simulink model "model"  (R2022a)
settings: Solver=VariableStepAuto  StartTime=0.0  StopTime=0.12  MaxStep=0.0001  RelTol=1e-3
values from neighbouring files (symbols this model uses):
  betta = Mp/wnom    (= 0.600343053173)    [config.m]
  J = J1+J2    (= 0.01)    [config.m]
  Kp = T1/(2*Tmu*Kpr*Kw)    [config.m]
  Kpr = 10    [config.m]
  Kw = u_zad/wnom    (= 0.0857632933105)    [config.m]
  Mc = 0    [config.m]    (also in tasks.m = Mc2)
  T1 = 1/T12(2)    [config.m]
  T2 = 1/T12(1)    [config.m]
  Te = 3.3/1000    (= 0.0033)    [config.m]
  Ti = T1    [config.m]
  Tm = J/betta    (= 0.0166571428571)    [config.m]
  Tmu = Tpr + T2    [config.m]
  Tpr = 0.5/1000    (= 0.0005)    [config.m]
  w_zad = wnom    (= 116.6)    [config.m]    (also in tasks.m = 0)
settings Model: Creator=Vvlad  LastModifiedBy=Vvlad

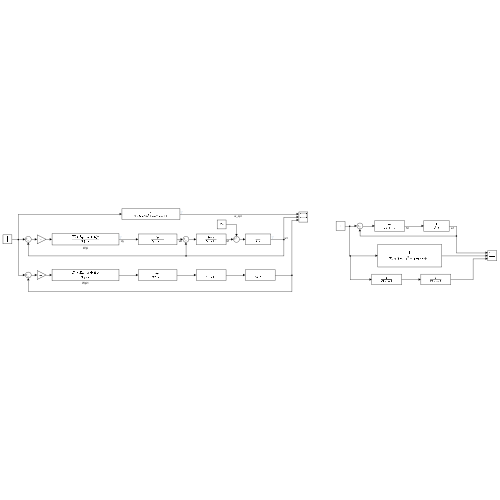
[thumbnail: Simulink's stored preview of the top-level diagram]
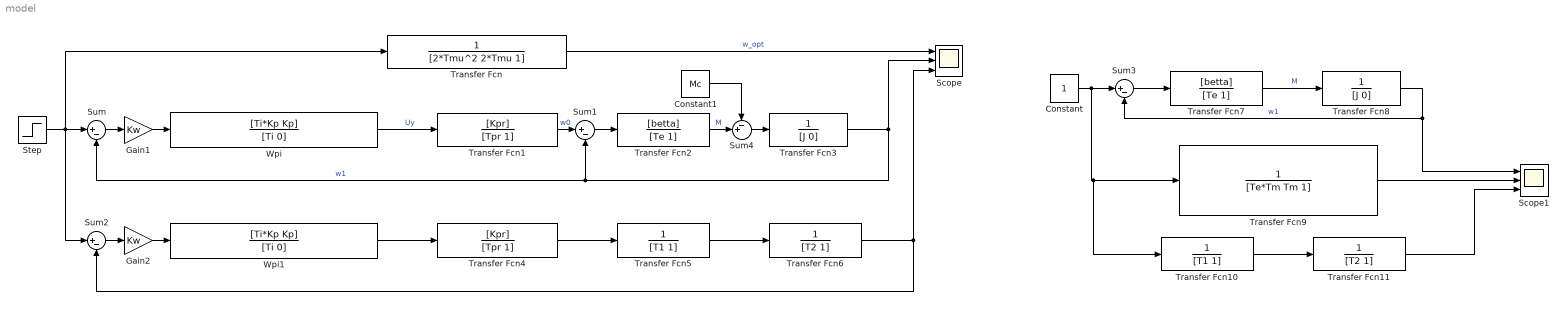
== system model ==
  Constant : Constant
  Constant1 : Constant  Value=Mc
  Gain1 : Gain  Gain=Kw
  Gain2 : Gain  Gain=Kw
  Scope : Scope  NumInputPorts=3
  Scope1 : Scope  NumInputPorts=3
  Step : Step  Time=0  After=w_zad  SampleTime=0
  Sum{,1..3} (4 alike) : Sum  Inputs=|+-
  Sum4 : Sum  Inputs=-+|
  Transfer Fcn : TransferFcn  Denominator=[2*Tmu^2 2*Tmu 1]
  Transfer Fcn1 : TransferFcn  Numerator=[Kpr]  Denominator=[Tpr 1]
  Transfer Fcn10 : TransferFcn  Denominator=[T1 1]
  Transfer Fcn11 : TransferFcn  Denominator=[T2 1]
  Transfer Fcn2 : TransferFcn  Numerator=[betta]  Denominator=[Te 1]
  Transfer Fcn3 : TransferFcn  Denominator=[J 0]
  Transfer Fcn4 : TransferFcn  Numerator=[Kpr]  Denominator=[Tpr 1]
  Transfer Fcn5 : TransferFcn  Denominator=[T1 1]
  Transfer Fcn6 : TransferFcn  Denominator=[T2 1]
  Transfer Fcn7 : TransferFcn  Numerator=[betta]  Denominator=[Te 1]
  Transfer Fcn8 : TransferFcn  Denominator=[J 0]
  Transfer Fcn9 : TransferFcn  Denominator=[Te*Tm Tm 1]
  Wpi : TransferFcn  Numerator=[Ti*Kp Kp]  Denominator=[Ti 0]
  Wpi1 : TransferFcn  Numerator=[Ti*Kp Kp]  Denominator=[Ti 0]
  wires:
  Transfer Fcn/1 -> Scope/1  "w_opt"
  Sum/1 -> Gain1/1
  Transfer Fcn2/1 -> Sum4/2  "M"
  Transfer Fcn1/1 -> Sum1/1  "w0"
  Wpi/1 -> Transfer Fcn1/1  "Uy"
  Step/1 -> Sum2/1, Sum/1, Transfer Fcn/1
  Transfer Fcn3/1 -> Sum1/2, Sum/2, Scope/2  "w1"
  Gain1/1 -> Wpi/1
  Gain2/1 -> Wpi1/1
  Sum2/1 -> Gain2/1
  Wpi1/1 -> Transfer Fcn4/1
  Transfer Fcn5/1 -> Transfer Fcn6/1
  Transfer Fcn4/1 -> Transfer Fcn5/1
  Transfer Fcn6/1 -> Sum2/2, Scope/3
  Sum1/1 -> Transfer Fcn2/1
  Constant/1 -> Transfer Fcn10/1, Transfer Fcn9/1, Sum3/1
  Sum3/1 -> Transfer Fcn7/1
  Transfer Fcn7/1 -> Transfer Fcn8/1  "M"
  Transfer Fcn8/1 -> Sum3/2, Scope1/1  "w1"
  Transfer Fcn9/1 -> Scope1/2
  Transfer Fcn10/1 -> Transfer Fcn11/1
  Transfer Fcn11/1 -> Scope1/3
  Sum4/1 -> Transfer Fcn3/1
  Constant1/1 -> Sum4/1
